simulink model "VDPOL"  (Simulink 10.0)
settings: Solver=ode45  StartTime=0.0  StopTime=2000  RelTol=1e-3  EnableMultiTasking=on
libraries: simulink x1
settings Model: Creator=UX31  LastModifiedBy=unknown
settings DataIOCC: LimitDataPoints=on
settings DebuggingCC: UnderspecifiedInitializationDetection=Simplified  MergeDetectMultiDrivingBlocksExec=error  SolverPrmCheckMsg=warning
settings GRTTargetCC: GeneratePreprocessorConditionals=Disable all  CombineOutputUpdateFcns=on  GRTInterface=off
settings ConfigComp: CovExternalEMLEnable=off  CovSFcnEnable=off

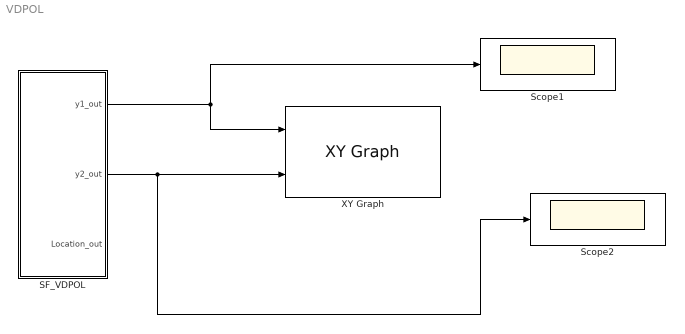
== system VDPOL ==
  SF_VDPOL : Stateflow chart  TreatAsAtomicUnit=on
  Scope1 : Scope
  Scope2 : Scope
  XY Graph : simulink/Sinks/XY Graph  xmin=-5  xmax=5  ymin=-6  ymax=6  st=-1
  wires:
  SF_VDPOL/1(y1_out) -> Scope1/1, XY Graph/1
  SF_VDPOL/2(y2_out) -> XY Graph/2, Scope2/1

== stateflow chart SF_VDPOL ==
  settings: updateMethod=CONTINUOUS
  state VDPOL
    du:
    y1_dot=y2;
    y2_dot=k*(1-y1^2)*y2-y1;
    y1_out=y1;
    y2_out=y2;
    Location_out =1;
  (default) -> VDPOL : {y1=2;y2=0}
  data: y1 local double; y1_out output double; y2 local double; y2_out output double; Location_out output double; k constant double =2
  data y1 settings: updateMethod=SF_CONTINUOUS_TIME_DATA
  data y2 settings: updateMethod=SF_CONTINUOUS_TIME_DATA
